simulink model "IA1_test"  (R2022b)
settings: Solver=VariableStepAuto  StartTime=0.0  StopTime=10.0  RelTol=1e-3
libraries: simulink x2, spsBistableLib x1
settings Model: Creator=Ccm  LastModifiedBy=Ccm

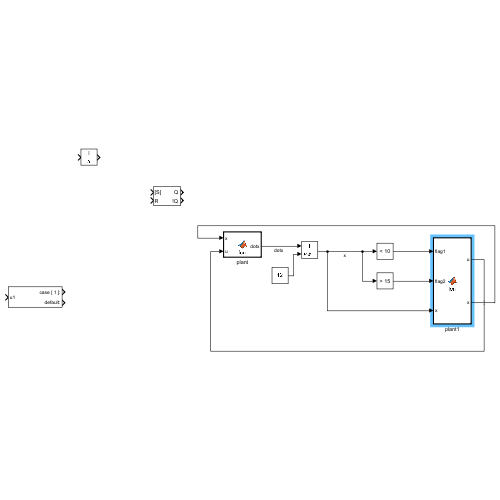
[thumbnail: Simulink's stored preview of the top-level diagram]
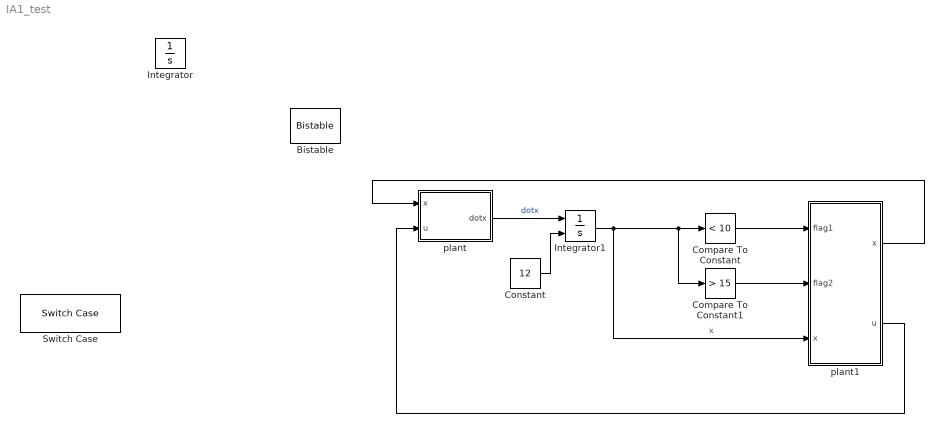
== system IA1_test ==
  Bistable : spsBistableLib/Bistable  Qpriority=Set  ic=0  Ts=0
      settings: LibrarySourceBlock=sps_lib/Control/Bistable
  Compare To Constant : simulink/Logic and Bit Operations/Compare To Constant  relop=<  const=10  OutDataTypeStr=boolean
  Compare To Constant1 : simulink/Logic and Bit Operations/Compare To Constant  relop=>  const=15  OutDataTypeStr=boolean
  Constant : Constant  Value=12
  Integrator : Integrator
  Integrator1 : Integrator  InitialConditionSource=external
  Switch Case : SwitchCase
  plant : MATLAB Function  TreatAsAtomicUnit=on
  plant1 : MATLAB Function  TreatAsAtomicUnit=on
  wires:
  plant/1(dotx) -> Integrator1/1  "dotx"
  Integrator1/1 -> Compare To Constant1/1, Compare To Constant/1, plant1/3("x ")  "x"
  Compare To Constant/1 -> plant1/1(flag1)
  Compare To Constant1/1 -> plant1/2(flag2)
  plant1/2(u) -> plant/2(u)
  plant1/1(x) -> plant/1(x)
  Constant/1 -> Integrator1/2

== matlab function IA1_test/plant ==
  data: x input; dotx output; u input
function dotx = fcn(x,u)

dotx = -x+u;

== matlab function IA1_test/plant1 ==
  data: x output; flag1 input; flag2 input; x input; u output
function [x,u] = fcn(flag1,flag2,x)

if flag1 >0
    x = x;
    u = 25;
if flag2 >0
    u = 0;
    x = x;
